simulink model "Task2simulink"  (R2021a)
settings: Solver=VariableStepAuto  StartTime=0.0  StopTime=10000  RelTol=1e-3
values from neighbouring files (symbols this model uses):
  K1 = 1/(C1*C2*R2)    (= 3.33333333333e-05)    [Task1.m]
  K2 = 1/(C1*R12)    (= 0.004)    [Task1.m]
  K3 = 1/(C2*R23)    (= 0.00333333333333)    [Task1.m]
  K4 = (R2^2-(R12*R23))/(C1*C2*R12*R23*R2^2)    (= 1e-05)    [Task1.m]
  P0 = 1/C1    (= 0.02)    [Task1.m]
  P1 = 1/(C1^2*R12)    (= 8e-05)    [Task1.m]
  P2 = 1/(C1*C2*R23)    (= 6.66666666667e-05)    [Task1.m]
  P3 = 1/(C1^2*C2*R12*R23)    (= 2.66666666667e-07)    [Task1.m]
  P4 = 2/(C1*R12)    (= 0.008)    [Task1.m]
  P5 = 1/(C2*R23)    (= 0.00333333333333)    [Task1.m]
  P6 = 1/(C1^2*R12^2)    (= 1.6e-05)    [Task1.m]
  P7 = 1/(C1*C2*R12*R23)    (= 1.33333333333e-05)    [Task1.m]
  P8 = (R2^2-R12*R23)/(C1*C2*R12*R23*R2^2)    (= 1e-05)    [Task1.m]
  P9 = (R2^2-(R12*R23))/(C1^2*C2*R12^2*R23*R2^2)    (= 4e-08)    [Task1.m]
settings Model: Creator=coa21ptl  LastModifiedBy=coa21ptl
settings DataIOCC: ReturnWorkspaceOutputs=off

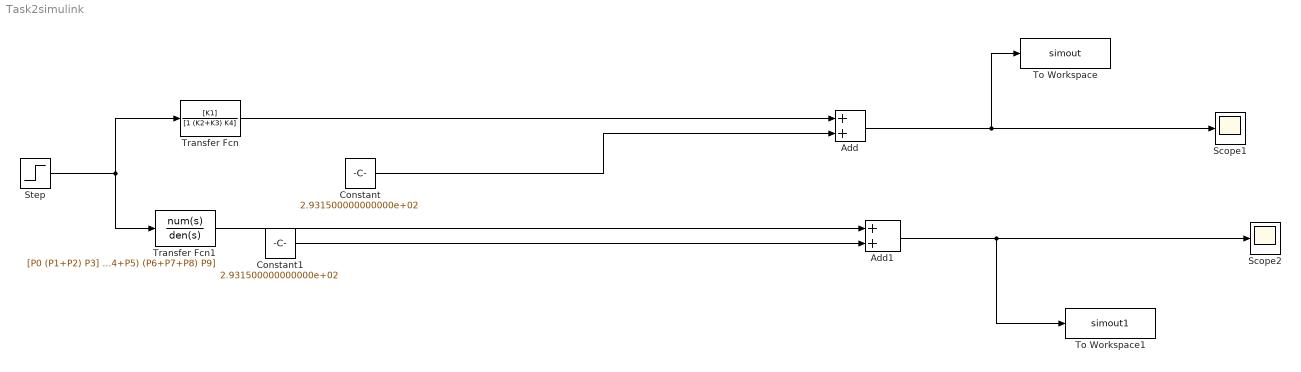
== system Task2simulink ==
  Add : Sum
  Add1 : Sum
  Constant : Constant  Value=2.931500000000000e+02
  Constant1 : Constant  Value=2.931500000000000e+02
  Scope1 : Scope
  Scope2 : Scope
  Step : Step  Time=600  After=3  SampleTime=0
  To Workspace : ToWorkspace  VariableName=simout  SaveFormat=Timeseries  SampleTime=-1
  To Workspace1 : ToWorkspace  VariableName=simout1  SaveFormat=Timeseries  SampleTime=-1
  Transfer Fcn : TransferFcn  Numerator=[K1]  Denominator=[1 (K2+K3) K4]
  Transfer Fcn1 : TransferFcn  Numerator=[P0 (P1+P2) P3]  Denominator=[1 (P4+P5) (P6+P7+P8) P9]
  wires:
  Step/1 -> Transfer Fcn1/1, Transfer Fcn/1
  Constant/1 -> Add/2
  Transfer Fcn/1 -> Add/1
  Constant1/1 -> Add1/2
  Add/1 -> To Workspace/1, Scope1/1
  Transfer Fcn1/1 -> Add1/1
  Add1/1 -> To Workspace1/1, Scope2/1
